simulink model "pwr_computeEnginePower"  (R2019b)
settings: Solver=FixedStepDiscrete  StartTime=0.0  StopTime=10.0  RelTol=1e-3
libraries: simulink x27
settings Model: Creator=vranken  LastModifiedBy=vranken
settings OptimizationCC: DefaultParameterBehavior=Inlined  EnhancedBackFolding=on  PassReuseOutputArgsAs=Individual arguments  ZeroExternalMemoryAtStartup=off  ZeroInternalMemoryAtStartup=off  OptimizeBlockOrder=speed  DifferentSizesBufferReuse=on  OptimizationCustomize=off  EfficientTunableParamExpr=on
settings DebuggingCC: ParameterTunabilityLossMsg=error
settings HardwareCC: ProdBitPerInt=16  ProdBitPerPointer=16  ProdBitPerSizeT=16  ProdBitPerPtrDiffT=16  ProdLargestAtomicFloat=None  ProdWordSize=8  ProdHWDeviceType=Atmel->AVR
settings SFSimCC: MATLABDynamicMemAlloc=off
settings RTWCC: SystemTargetFile=ert.tlc  GenCodeOnly=on  TemplateMakefile=ert_default_tmf  GenerateReport=on  IncludeHyperlinkInReport=on  LaunchReport=on  GenerateTraceInfo=on  GenerateTraceReport=on  GenerateTraceReportSl=on  GenerateTraceReportSf=on  GenerateTraceReportEml=on
settings CodeAppCC: ForceParamTrailComments=on  IgnoreCustomStorageClasses=off  OperatorAnnotations=on  SimulinkDataObjDesc=on  SFDataObjDesc=on  InsertBlockDesc=on
settings ERTTargetCC: TargetLangStandard=C99 (ISO)  SupportAbsoluteTime=off  PurelyIntegerCode=on  SupportNonFinite=off  SupportComplex=off  GenerateASAP2=on  InlinedParameterPlacement=NonHierarchical  ERTCustomFileTemplate=example_file_process.tlc  IndentStyle=Allman  IndentSize=4

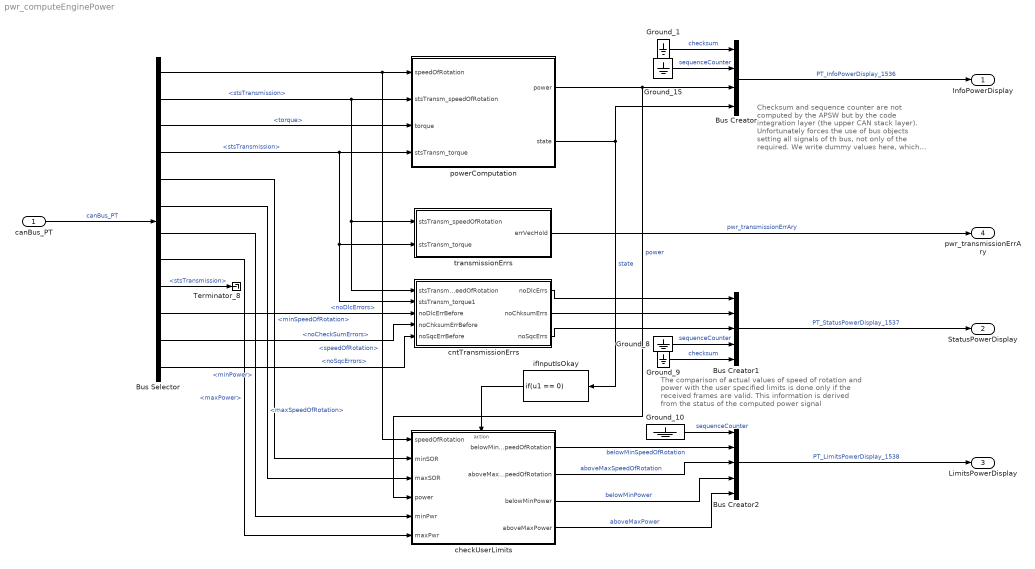
== system pwr_computeEnginePower ==
  note: The comparison of actual values of speed of rotation
      |  and power with the user specified limits is done only
      | if the received frames are valid. This information is
      | derived from the status of the computed power signal
  note: Checksum and sequence counter are not
      | computed by the APSW but by the code
      | integration layer (the upper CAN stack layer).
      | Unfortunately forces the use of bus objects
      | setting all signals of th bus, not only of
      | the required. We write dummy values here,
      | which will be overwritten by the CAN stack
  canBus_PT : Inport  OutDataTypeStr=Bus: cap_canBus_PT_t  BusOutputAsStruct=on
  Bus Creator : BusCreator  Inputs=4  OutDataTypeStr=Bus: cap_PT_InfoPowerDisplay_1536_t  NonVirtualBus=on
  Bus Creator1 : BusCreator  Inputs=5  OutDataTypeStr=Bus: cap_PT_StatusPowerDisplay_1537_t  NonVirtualBus=on
  Bus Creator2 : BusCreator  Inputs=5  OutDataTypeStr=Bus: cap_PT_LimitsPowerDisplay_1538_t  NonVirtualBus=on
  Bus Selector : BusSelector  OutputSignals=PT_StateEcu01_1024_sts.signals.speedOfRotation,PT_StateEcu01_1024_sts.stsTransmission,PT_StateEcu02_1040_sts.signals.torque,PT_StateEcu02_1040_sts.stsTransmission,PT_UserLimits_2032_sts.signals.minSpeedOfRotation,PT_UserLimits_2032_sts.signals.maxSpeedOfRotation,PT_UserLimits_2032_sts.signals.minPower,PT_UserLimits_2032_sts.signals.maxPower,PT_UserLimits_2032_sts.stsTransmission,PT_StatusPowerDisplay_1537_sts.signals.noDlcErrors,PT_StatusPowerDisplay_1537_sts.signals.noCheckSumErrors,PT_StatusPowerDisplay_1537_sts.signals.noSqcErrors
  Ground_{1,8..10,15} (5 alike) : Ground
  Terminator_8 : Terminator
  checkUserLimits : Subsystem  TreatAsAtomicUnit=on  RTWFcnName=pwr_detectAndCountError
      settings: RTWFcnNameOpts=User specified
  cntTransmissionErrs : Subsystem
  ifInputIsOkay : If  IfExpression=u1 == 0  ShowElse=off
  powerComputation : Subsystem
  transmissionErrs : Subsystem
  InfoPowerDisplay : Outport  OutDataTypeStr=Bus: cap_PT_InfoPowerDisplay_1536_t
  StatusPowerDisplay : Outport  Port=2  OutDataTypeStr=Bus: cap_PT_StatusPowerDisplay_1537_t
  LimitsPowerDisplay : Outport  Port=3  OutDataTypeStr=Bus: cap_PT_LimitsPowerDisplay_1538_t
  pwr_transmissionErrAry : Outport  Port=4
  wires:
  Bus Creator1/1 -> StatusPowerDisplay/1  "PT_StatusPowerDisplay_1537"
  Ground_15/1 -> Bus Creator/2  "sequenceCounter"
  Bus Selector/8 -> checkUserLimits/6(maxPwr)  "<maxPower>"
  Bus Selector/10 -> cntTransmissionErrs/3(noDlcErrBefore)  "<noDlcErrors>"
  Bus Selector/9 -> Terminator_8/1  "<stsTransmission>"
  Bus Selector/7 -> checkUserLimits/5(minPwr)  "<minPower>"
  powerComputation/1(power) -> Bus Creator/3, checkUserLimits/4(power)  "power"
  canBus_PT/1 -> Bus Selector/1  "canBus_PT"
  Bus Selector/6 -> checkUserLimits/3(maxSOR)  "<maxSpeedOfRotation>"
  powerComputation/2(state) -> Bus Creator/4, ifInputIsOkay/1  "state"
  cntTransmissionErrs/2(noChksumErrs) -> Bus Creator1/2
  ifInputIsOkay/1 -> checkUserLimits/Action
  Bus Selector/11 -> cntTransmissionErrs/4(noChksumErrBefore)  "<noCheckSumErrors>"
  Bus Selector/5 -> checkUserLimits/2(minSOR)  "<minSpeedOfRotation>"
  transmissionErrs/1(errVecHold) -> pwr_transmissionErrAry/1  "pwr_transmissionErrAry"
  Ground_1/1 -> Bus Creator/1  "checksum"
  checkUserLimits/4(aboveMaxPower) -> Bus Creator2/5  "aboveMaxPower"
  Bus Creator2/1 -> LimitsPowerDisplay/1  "PT_LimitsPowerDisplay_1538"
  cntTransmissionErrs/3(noSqcErrs) -> Bus Creator1/3
  Bus Selector/4 -> powerComputation/4(stsTransm_torque), cntTransmissionErrs/2(stsTransm_torque1), transmissionErrs/2(stsTransm_torque)  "<stsTransmission>"
  checkUserLimits/3(belowMinPower) -> Bus Creator2/4  "belowMinPower"
  Ground_9/1 -> Bus Creator1/5  "checksum"
  Bus Selector/1 -> powerComputation/1(speedOfRotation), checkUserLimits/1(speedOfRotation)  "<speedOfRotation>"
  checkUserLimits/2(aboveMaxSpeedOfRotation) -> Bus Creator2/3  "aboveMaxSpeedOfRotation"
  Bus Selector/3 -> powerComputation/3(torque)  "<torque>"
  cntTransmissionErrs/1(noDlcErrs) -> Bus Creator1/1
  Bus Selector/12 -> cntTransmissionErrs/5(noSqcErrBefore)  "<noSqcErrors>"
  Bus Selector/2 -> powerComputation/2(stsTransm_speedOfRotation), cntTransmissionErrs/1(stsTransm_speedOfRotation), transmissionErrs/1(stsTransm_speedOfRotation)  "<stsTransmission>"
  checkUserLimits/1(belowMinSpeedOfRotation) -> Bus Creator2/2  "belowMinSpeedOfRotation"
  Bus Creator/1 -> InfoPowerDisplay/1  "PT_InfoPowerDisplay_1536"
  Ground_8/1 -> Bus Creator1/4  "sequenceCounter"
  Ground_10/1 -> Bus Creator2/1  "sequenceCounter"

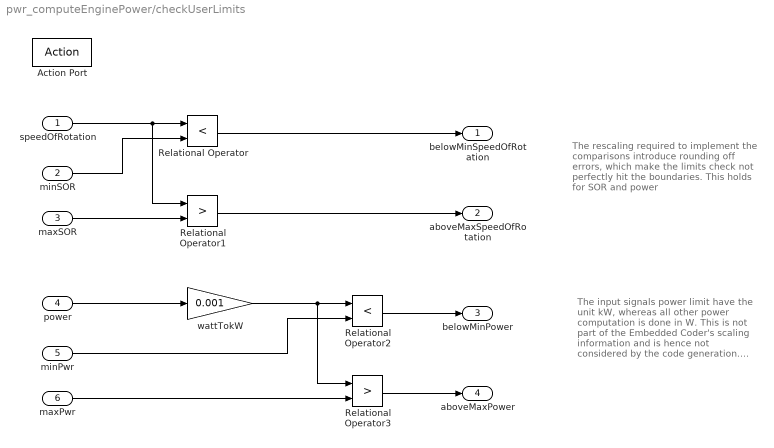
== system pwr_computeEnginePower/checkUserLimits ==
  note: The input signals power limit
      | have the unit kW, whereas all other
      | power computation is done in W.
      | This is not part of the Embedded
      | Coder's scaling information and is
      | hence not considered by the code
      | generation. We need to perform
      | this kind of rescaling by an explicit
      | multiplication operation
  note: The rescaling required to implement
      | the comparisons introduce rounding
      | off errors, which make the limits check
      | not perfectly hit the boundaries. This
      | holds for SOR and power
  speedOfRotation : Inport
  minSOR : Inport  Port=2
  maxSOR : Inport  Port=3
  power : Inport  Port=4
  minPwr : Inport  Port=5
  maxPwr : Inport  Port=6
  Action Port : ActionPort  PropagateVarSize=During execution  ActionPortLabel=if(u1 == 0)
  Relational Operator : RelationalOperator  Operator=<  OutDataTypeStr=boolean  RndMeth=Nearest
  Relational Operator1 : RelationalOperator  Operator=>  OutDataTypeStr=boolean  RndMeth=Nearest
  Relational Operator2 : RelationalOperator  Operator=<  OutDataTypeStr=boolean  RndMeth=Nearest
  Relational Operator3 : RelationalOperator  Operator=>  OutDataTypeStr=boolean  RndMeth=Nearest
  wattTokW : Gain  Gain=0.001  OutDataTypeStr=fixdt(0,16,2^-1,-10)
  belowMinSpeedOfRotation : Outport
  aboveMaxSpeedOfRotation : Outport  Port=2
  belowMinPower : Outport  Port=3
  aboveMaxPower : Outport  Port=4
  wires:
  speedOfRotation/1 -> Relational Operator/1, Relational Operator1/1
  minSOR/1 -> Relational Operator/2
  Relational Operator/1 -> belowMinSpeedOfRotation/1
  maxSOR/1 -> Relational Operator1/2
  Relational Operator1/1 -> aboveMaxSpeedOfRotation/1
  power/1 -> wattTokW/1
  minPwr/1 -> Relational Operator2/2
  Relational Operator2/1 -> belowMinPower/1
  maxPwr/1 -> Relational Operator3/2
  Relational Operator3/1 -> aboveMaxPower/1
  wattTokW/1 -> Relational Operator2/1, Relational Operator3/1

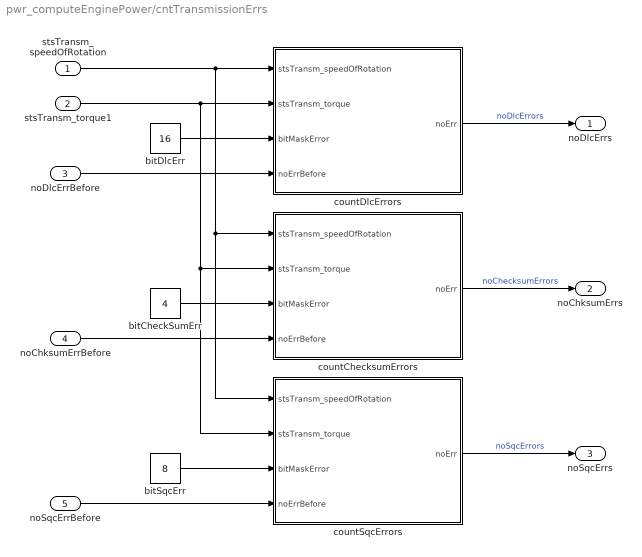
== system pwr_computeEnginePower/cntTransmissionErrs ==
  stsTransm_speedOfRotation : Inport
  stsTransm_torque1 : Inport  Port=2
  noDlcErrBefore : Inport  Port=3
  noChksumErrBefore : Inport  Port=4
  noSqcErrBefore : Inport  Port=5
  bitCheckSumErr : Constant  Value=4  OutDataTypeStr=uint8
  bitDlcErr : Constant  Value=16  OutDataTypeStr=uint8
  bitSqcErr : Constant  Value=8  OutDataTypeStr=uint8
  countChecksumErrors : Subsystem  TreatAsAtomicUnit=on  RTWFcnName=pwr_detectAndCountError
      settings: RTWFcnNameOpts=User specified
  countDlcErrors : Subsystem  TreatAsAtomicUnit=on  RTWFcnName=pwr_detectAndCountError
      settings: RTWFcnNameOpts=User specified
  countSqcErrors : Subsystem  TreatAsAtomicUnit=on  RTWFcnName=pwr_detectAndCountError
      settings: RTWFcnNameOpts=User specified
  noDlcErrs : Outport
  noChksumErrs : Outport  Port=2
  noSqcErrs : Outport  Port=3
  wires:
  bitDlcErr/1 -> countDlcErrors/3(bitMaskError)
  bitCheckSumErr/1 -> countChecksumErrors/3(bitMaskError)
  bitSqcErr/1 -> countSqcErrors/3(bitMaskError)
  stsTransm_speedOfRotation/1 -> countDlcErrors/1(stsTransm_speedOfRotation), countChecksumErrors/1(stsTransm_speedOfRotation), countSqcErrors/1(stsTransm_speedOfRotation)
  stsTransm_torque1/1 -> countDlcErrors/2(stsTransm_torque), countChecksumErrors/2(stsTransm_torque), countSqcErrors/2(stsTransm_torque)
  countDlcErrors/1(noErr) -> noDlcErrs/1  "noDlcErrors"
  noDlcErrBefore/1 -> countDlcErrors/4(noErrBefore)
  countChecksumErrors/1(noErr) -> noChksumErrs/1  "noChecksumErrors"
  noChksumErrBefore/1 -> countChecksumErrors/4(noErrBefore)
  countSqcErrors/1(noErr) -> noSqcErrs/1  "noSqcErrors"
  noSqcErrBefore/1 -> countSqcErrors/4(noErrBefore)

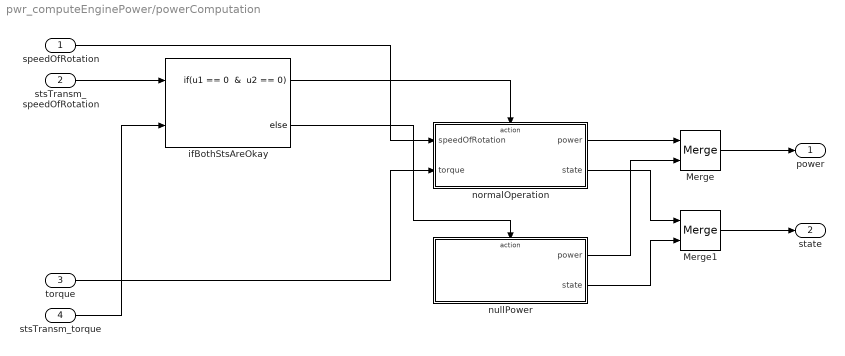
== system pwr_computeEnginePower/powerComputation ==
  speedOfRotation : Inport
  stsTransm_speedOfRotation : Inport  Port=2
  torque : Inport  Port=3
  stsTransm_torque : Inport  Port=4
  Merge : Merge
  Merge1 : Merge
  ifBothStsAreOkay : If  NumInputs=2  IfExpression="u1 == 0  &  u2 == 0"
  normalOperation : Subsystem  TreatAsAtomicUnit=on
  nullPower : Subsystem  TreatAsAtomicUnit=on
  power : Outport
  state : Outport  Port=2
  wires:
  speedOfRotation/1 -> normalOperation/1(speedOfRotation)
  stsTransm_speedOfRotation/1 -> ifBothStsAreOkay/1
  stsTransm_torque/1 -> ifBothStsAreOkay/2
  ifBothStsAreOkay/1 -> normalOperation/Action
  torque/1 -> normalOperation/2(torque)
  ifBothStsAreOkay/2 -> nullPower/Action
  normalOperation/1(power) -> Merge/1
  nullPower/1(power) -> Merge/2
  normalOperation/2(state) -> Merge1/1
  nullPower/2(state) -> Merge1/2
  Merge/1 -> power/1
  Merge1/1 -> state/1

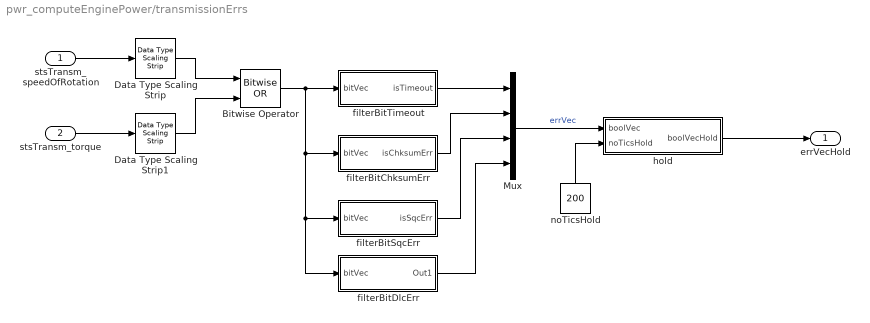
== system pwr_computeEnginePower/transmissionErrs ==
  stsTransm_speedOfRotation : Inport
  stsTransm_torque : Inport  Port=2
  Bitwise Operator : simulink/Logic and Bit Operations/Bitwise Operator  logicop=OR  UseBitMask=off  NumInputPorts=2  BitMask=bin2dec('11011001')  BitMaskRealWorld=Stored Integer
  Data Type Scaling Strip : simulink/Signal Attributes/Data Type Scaling Strip
      settings: SourceProductName=Simulink  SourceProductBaseCode=SL
  Data Type Scaling Strip1 : simulink/Signal Attributes/Data Type Scaling Strip
      settings: SourceProductName=Simulink  SourceProductBaseCode=SL
  Mux : Mux
  filterBitChksumErr : Subsystem
  filterBitDlcErr : Subsystem
  filterBitSqcErr : Subsystem
  filterBitTimeout : Subsystem
  hold : Subsystem
  noTicsHold : Constant  Value=200  OutDataTypeStr=uint8
  errVecHold : Outport
  wires:
  stsTransm_speedOfRotation/1 -> Data Type Scaling Strip/1
  stsTransm_torque/1 -> Data Type Scaling Strip1/1
  Data Type Scaling Strip/1 -> Bitwise Operator/1
  Mux/1 -> hold/1(boolVec)  "errVec"
  Data Type Scaling Strip1/1 -> Bitwise Operator/2
  Bitwise Operator/1 -> filterBitSqcErr/1(bitVec), filterBitDlcErr/1(bitVec), filterBitChksumErr/1(bitVec), filterBitTimeout/1(bitVec)
  filterBitChksumErr/1(isChksumErr) -> Mux/2
  filterBitSqcErr/1(isSqcErr) -> Mux/3
  filterBitDlcErr/1(Out1) -> Mux/4
  filterBitTimeout/1(isTimeout) -> Mux/1
  hold/1(boolVecHold) -> errVecHold/1
  noTicsHold/1 -> hold/2(noTicsHold)

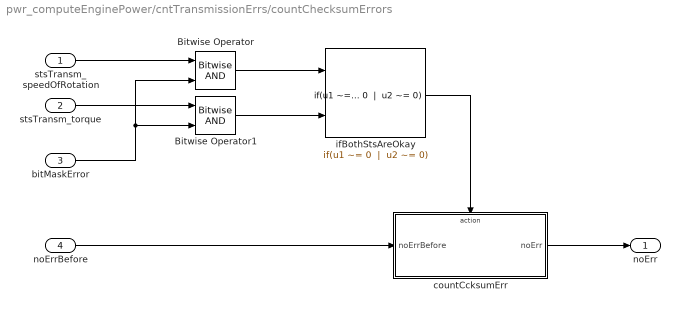
== system pwr_computeEnginePower/cntTransmissionErrs/countChecksumErrors ==
  stsTransm_speedOfRotation : Inport
  stsTransm_torque : Inport  Port=2
  bitMaskError : Inport  Port=3
  noErrBefore : Inport  Port=4
  Bitwise Operator : simulink/Logic and Bit Operations/Bitwise Operator  logicop=AND  UseBitMask=off  NumInputPorts=2  BitMask=bin2dec('11011001')  BitMaskRealWorld=Stored Integer
  Bitwise Operator1 : simulink/Logic and Bit Operations/Bitwise Operator  logicop=AND  UseBitMask=off  NumInputPorts=2  BitMask=bin2dec('11011001')  BitMaskRealWorld=Stored Integer
  countCcksumErr : Subsystem  TreatAsAtomicUnit=on
  ifBothStsAreOkay : If  NumInputs=2  IfExpression="u1 ~= 0  |  u2 ~= 0"  ShowElse=off
  noErr : Outport
  wires:
  ifBothStsAreOkay/1 -> countCcksumErr/Action
  stsTransm_torque/1 -> Bitwise Operator1/1
  stsTransm_speedOfRotation/1 -> Bitwise Operator/1
  noErrBefore/1 -> countCcksumErr/1(noErrBefore)
  countCcksumErr/1(noErr) -> noErr/1
  bitMaskError/1 -> Bitwise Operator/2, Bitwise Operator1/2
  Bitwise Operator/1 -> ifBothStsAreOkay/1
  Bitwise Operator1/1 -> ifBothStsAreOkay/2

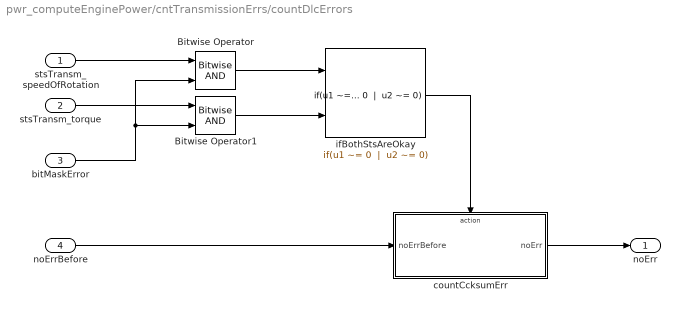
== system pwr_computeEnginePower/cntTransmissionErrs/countDlcErrors ==
  stsTransm_speedOfRotation : Inport
  stsTransm_torque : Inport  Port=2
  bitMaskError : Inport  Port=3
  noErrBefore : Inport  Port=4
  Bitwise Operator : simulink/Logic and Bit Operations/Bitwise Operator  logicop=AND  UseBitMask=off  NumInputPorts=2  BitMask=bin2dec('11011001')  BitMaskRealWorld=Stored Integer
  Bitwise Operator1 : simulink/Logic and Bit Operations/Bitwise Operator  logicop=AND  UseBitMask=off  NumInputPorts=2  BitMask=bin2dec('11011001')  BitMaskRealWorld=Stored Integer
  countCcksumErr : Subsystem  TreatAsAtomicUnit=on
  ifBothStsAreOkay : If  NumInputs=2  IfExpression="u1 ~= 0  |  u2 ~= 0"  ShowElse=off
  noErr : Outport
  wires:
  ifBothStsAreOkay/1 -> countCcksumErr/Action
  stsTransm_torque/1 -> Bitwise Operator1/1
  stsTransm_speedOfRotation/1 -> Bitwise Operator/1
  noErrBefore/1 -> countCcksumErr/1(noErrBefore)
  countCcksumErr/1(noErr) -> noErr/1
  bitMaskError/1 -> Bitwise Operator/2, Bitwise Operator1/2
  Bitwise Operator/1 -> ifBothStsAreOkay/1
  Bitwise Operator1/1 -> ifBothStsAreOkay/2

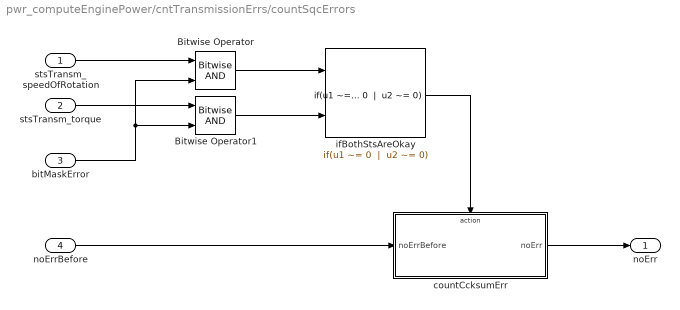
== system pwr_computeEnginePower/cntTransmissionErrs/countSqcErrors ==
  stsTransm_speedOfRotation : Inport
  stsTransm_torque : Inport  Port=2
  bitMaskError : Inport  Port=3
  noErrBefore : Inport  Port=4
  Bitwise Operator : simulink/Logic and Bit Operations/Bitwise Operator  logicop=AND  UseBitMask=off  NumInputPorts=2  BitMask=bin2dec('11011001')  BitMaskRealWorld=Stored Integer
  Bitwise Operator1 : simulink/Logic and Bit Operations/Bitwise Operator  logicop=AND  UseBitMask=off  NumInputPorts=2  BitMask=bin2dec('11011001')  BitMaskRealWorld=Stored Integer
  countCcksumErr : Subsystem  TreatAsAtomicUnit=on
  ifBothStsAreOkay : If  NumInputs=2  IfExpression="u1 ~= 0  |  u2 ~= 0"  ShowElse=off
  noErr : Outport
  wires:
  Bitwise Operator1/1 -> ifBothStsAreOkay/2
  Bitwise Operator/1 -> ifBothStsAreOkay/1
  bitMaskError/1 -> Bitwise Operator1/2, Bitwise Operator/2
  countCcksumErr/1(noErr) -> noErr/1
  noErrBefore/1 -> countCcksumErr/1(noErrBefore)
  stsTransm_speedOfRotation/1 -> Bitwise Operator/1
  stsTransm_torque/1 -> Bitwise Operator1/1
  ifBothStsAreOkay/1 -> countCcksumErr/Action

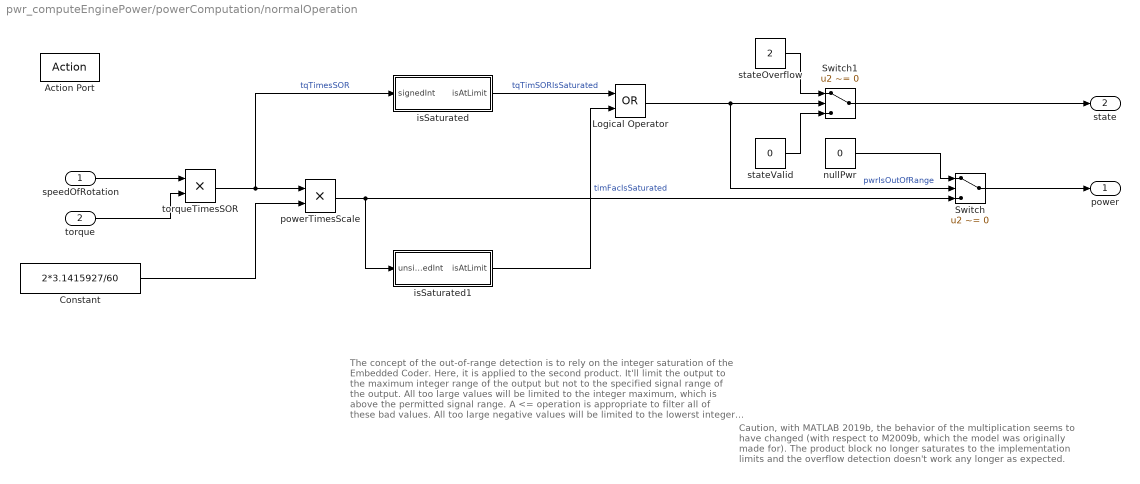
== system pwr_computeEnginePower/powerComputation/normalOperation ==
  note: Caution, with MATLAB 2019b, the behavior of the multiplication seems
      | to have changed (with respect to M2009b, which the model was
      | originally made for). The product block no longer saturates to the
      | implementation limits and the overflow detection doesn't work any
      | longer as expected.
  note: The concept of the out-of-range detection is to rely on the integer saturation
      | of the Embedded Coder. Here, it is applied to the second product. It'll limit
      | the output to the maximum integer range of the output but not to the specified
      | signal range of the output.
      |   All too large values will be limited to the integer maximum, which is above
      | the permitted signal range. A <= operation is appropriate to filter all of these
      | bad values.
      |   All too large negative values will be limited to the lowerst integer value, which
      | is the minimum permitted signal value at the same time. It's a binary zero. We
      | can't distinguish between a good but extreme value or a limited one if we see
      | the binary zero. This is ignored; binary zero is always considered a bad value.
      | Our logic effectively decreases the output signal range by one unit.
      |   A perfect out-of-range detection is nearly impossible in fixed point
      | computation since it requires some insight into the product operation. This
      | insight does the EC have during code generation but we don't have it on the
      | Simulink level.
      |  The best compromise would be the rule to never include the largest and
      | lowest integer values in the permitted signal range - then a safe detection
      | becomes possible in the way we present it here
  speedOfRotation : Inport
  torque : Inport  Port=2
  Action Port : ActionPort  PropagateVarSize=During execution  ActionPortLabel="if(u1 == 0  &  u2 == 0)"
  Constant : Constant  Value=2*3.1415927/60  OutDataTypeStr=fixdt(0,16,19)
  Logical Operator : Logic  Operator=OR  AllPortsSameDT=off  OutDataTypeStr=boolean
  Switch : Switch  Criteria=u2 ~= 0  OutDataTypeStr=Inherit: Inherit via back propagation
  Switch1 : Switch  Criteria=u2 ~= 0  OutDataTypeStr=Inherit: Inherit via back propagation
  isSaturated : Subsystem
  isSaturated1 : Subsystem
  nullPwr : Constant  Value=0  OutDataTypeStr=Inherit: Inherit via back propagation
  powerTimesScale : Product  OutDataTypeStr=fixdt(0,16,2^5,-500000)  RndMeth=Simplest  SaturateOnIntegerOverflow=on
  stateOverflow : Constant  Value=2  OutDataTypeStr=uint8
  stateValid : Constant  Value=0  OutDataTypeStr=uint8
  torqueTimesSOR : Product  OutMin=6553.5*(-500)  OutMax=6553.5*500  OutDataTypeStr=fixdt(1,32,9)  RndMeth=Simplest  SaturateOnIntegerOverflow=on
  power : Outport  InitialOutput=0
  state : Outport  Port=2  InitialOutput=1
  wires:
  speedOfRotation/1 -> torqueTimesSOR/1
  torque/1 -> torqueTimesSOR/2
  Constant/1 -> powerTimesScale/2
  powerTimesScale/1 -> isSaturated1/1(unsignedInt), Switch/3
  Switch/1 -> power/1
  Logical Operator/1 -> Switch1/2, Switch/2  "pwrIsOutOfRange"
  stateOverflow/1 -> Switch1/1
  stateValid/1 -> Switch1/3
  Switch1/1 -> state/1
  torqueTimesSOR/1 -> powerTimesScale/1, isSaturated/1(signedInt)  "tqTimesSOR"
  isSaturated/1(isAtLimit) -> Logical Operator/1  "tqTimSORIsSaturated"
  isSaturated1/1(isAtLimit) -> Logical Operator/2  "timFacIsSaturated"
  nullPwr/1 -> Switch/1

== system pwr_computeEnginePower/powerComputation/nullPower ==
  Action Port : ActionPort  PropagateVarSize=During execution  ActionPortLabel=else
  Constant : Constant  Value=0  OutDataTypeStr=Inherit: Inherit via back propagation
  stateInvalidInput : Constant  OutDataTypeStr=uint8
  power : Outport  InitialOutput=0
  state : Outport  Port=2  InitialOutput=1
  wires:
  Constant/1 -> power/1
  stateInvalidInput/1 -> state/1

== system pwr_computeEnginePower/transmissionErrs/filterBitChksumErr ==
  bitVec : Inport
  Compare To Zero : simulink/Logic and Bit Operations/Compare To Zero  relop=~=  OutDataTypeStr=boolean  ZeroCross=off
  andBitChksumErr : simulink/Logic and Bit Operations/Bitwise Operator  logicop=AND  UseBitMask=on  BitMask=4  BitMaskRealWorld=Stored Integer
  isChksumErr : Outport
  wires:
  bitVec/1 -> andBitChksumErr/1
  andBitChksumErr/1 -> Compare To Zero/1
  Compare To Zero/1 -> isChksumErr/1  "isChksumErr"

== system pwr_computeEnginePower/transmissionErrs/filterBitDlcErr ==
  bitVec : Inport
  Compare To Zero : simulink/Logic and Bit Operations/Compare To Zero  relop=~=  OutDataTypeStr=boolean  ZeroCross=off
  andBitDlcErr : simulink/Logic and Bit Operations/Bitwise Operator  logicop=AND  UseBitMask=on  BitMask=16  BitMaskRealWorld=Stored Integer
  Out1 : Outport
  wires:
  bitVec/1 -> andBitDlcErr/1
  andBitDlcErr/1 -> Compare To Zero/1
  Compare To Zero/1 -> Out1/1  "isDlcErr"

== system pwr_computeEnginePower/transmissionErrs/filterBitSqcErr ==
  note: isSqcErr
  bitVec : Inport
  Compare To Zero : simulink/Logic and Bit Operations/Compare To Zero  relop=~=  OutDataTypeStr=boolean  ZeroCross=off
  andBitSqcErr : simulink/Logic and Bit Operations/Bitwise Operator  logicop=AND  UseBitMask=on  BitMask=8  BitMaskRealWorld=Stored Integer
  isSqcErr : Outport
  wires:
  bitVec/1 -> andBitSqcErr/1
  andBitSqcErr/1 -> Compare To Zero/1
  Compare To Zero/1 -> isSqcErr/1

== system pwr_computeEnginePower/transmissionErrs/filterBitTimeout ==
  bitVec : Inport
  Compare To Zero : simulink/Logic and Bit Operations/Compare To Zero  relop=~=  OutDataTypeStr=boolean  ZeroCross=off
  andBitTimeout : simulink/Logic and Bit Operations/Bitwise Operator  logicop=AND  UseBitMask=on  BitMask=2  BitMaskRealWorld=Stored Integer
  isTimeout : Outport
  wires:
  andBitTimeout/1 -> Compare To Zero/1  "errTimeout"
  bitVec/1 -> andBitTimeout/1
  Compare To Zero/1 -> isTimeout/1  "isTimeout"

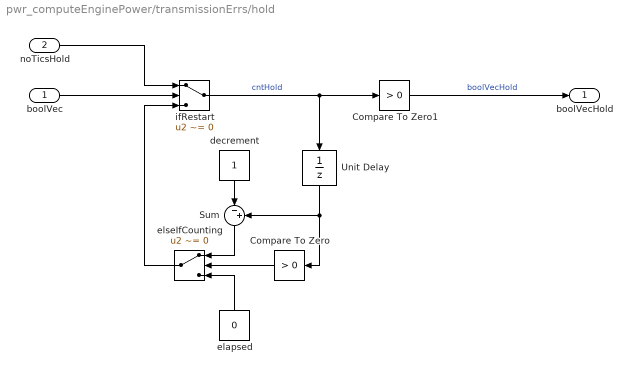
== system pwr_computeEnginePower/transmissionErrs/hold ==
  boolVec : Inport
  noTicsHold : Inport  Port=2
  Compare To Zero : simulink/Logic and Bit Operations/Compare To Zero  relop=>  OutDataTypeStr=boolean  ZeroCross=off
  Compare To Zero1 : simulink/Logic and Bit Operations/Compare To Zero  relop=>  OutDataTypeStr=boolean  ZeroCross=off
  Sum : Sum  Inputs=|-+
  Unit Delay : UnitDelay  SampleTime=-1
  decrement : Constant  OutDataTypeStr=uint8
  elapsed : Constant  Value=0  OutDataTypeStr=uint8
  elseIfCounting : Switch  Criteria=u2 ~= 0
  ifRestart : Switch  Criteria=u2 ~= 0
  boolVecHold : Outport
  wires:
  noTicsHold/1 -> ifRestart/1
  Unit Delay/1 -> Sum/2, Compare To Zero/1
  Sum/1 -> elseIfCounting/1
  decrement/1 -> Sum/1
  elapsed/1 -> elseIfCounting/3
  ifRestart/1 -> Unit Delay/1, Compare To Zero1/1  "cntHold"
  elseIfCounting/1 -> ifRestart/3
  Compare To Zero/1 -> elseIfCounting/2
  Compare To Zero1/1 -> boolVecHold/1  "boolVecHold"
  boolVec/1 -> ifRestart/2

== system pwr_computeEnginePower/cntTransmissionErrs/countChecksumErrors/countCcksumErr ==
  noErrBefore : Inport
  Action Port : ActionPort  PropagateVarSize=During execution  ActionPortLabel="if(u1 ~= 0  |  u2 ~= 0)"
  Sum : Sum  Inputs=|++
  increment : Constant  OutDataTypeStr=uint8
  noErr : Outport
  wires:
  noErrBefore/1 -> Sum/1
  Sum/1 -> noErr/1  "noChecksumErrors"
  increment/1 -> Sum/2

== system pwr_computeEnginePower/cntTransmissionErrs/countDlcErrors/countCcksumErr ==
  noErrBefore : Inport
  Action Port : ActionPort  PropagateVarSize=During execution  ActionPortLabel="if(u1 ~= 0  |  u2 ~= 0)"
  Sum : Sum  Inputs=|++
  increment : Constant  OutDataTypeStr=uint8
  noErr : Outport
  wires:
  noErrBefore/1 -> Sum/1
  Sum/1 -> noErr/1  "noDlcErrors"
  increment/1 -> Sum/2

== system pwr_computeEnginePower/cntTransmissionErrs/countSqcErrors/countCcksumErr ==
  noErrBefore : Inport
  Action Port : ActionPort  PropagateVarSize=During execution  ActionPortLabel="if(u1 ~= 0  |  u2 ~= 0)"
  Sum : Sum  Inputs=|++
  increment : Constant  OutDataTypeStr=uint8
  noErr : Outport
  wires:
  increment/1 -> Sum/2
  Sum/1 -> noErr/1  "noSqcErrors"
  noErrBefore/1 -> Sum/1

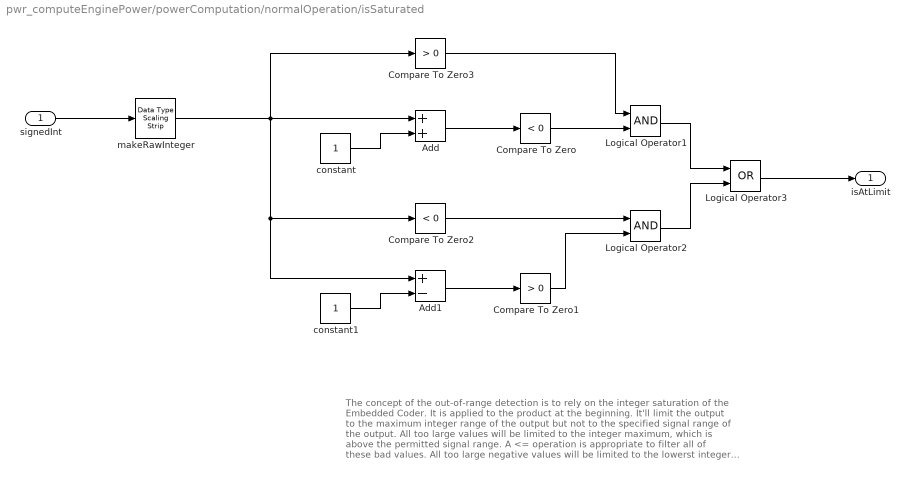
== system pwr_computeEnginePower/powerComputation/normalOperation/isSaturated ==
  note: The concept of the out-of-range detection is to rely on the integer saturation
      | of the Embedded Coder. It is applied to the product at the beginning. It'll limit
      | the output to the maximum integer range of the output but not to the specified
      | signal range of the output.
      |   All too large values will be limited to the integer maximum, which is above
      | the permitted signal range. A <= operation is appropriate to filter all of these
      | bad values.
      |   All too large negative values will be limited to the lowerst integer value, which
      | is the minimum permitted signal value at the same time. It's a binary zero. We
      | can't distinguish between a good but extreme value or a limited one if we see
      | the binary zero. This is ignored; binary zero is always considered a bad value.
      | Our logic effectively decreases the output signal range by one unit.
      |   A perfect out-of-range detection is nearly impossible in fixed point
      | computation since it requires some insight into the product operation. This
      | insight does the EC have during code generation but we don't have it on the
      | Simulink level.
      |  The best compromise would be the rule to never include the largest and
      | lowest integer values in the permitted signal range - then a safe detection
      | becomes possible in the way we present it here
  signedInt : Inport
  Add : Sum  OutDataTypeStr=Inherit: Same as accumulator  RndMeth=Simplest
  Add1 : Sum  Inputs=+-  OutDataTypeStr=Inherit: Same as accumulator  RndMeth=Simplest
  Compare To Zero : simulink/Logic and Bit Operations/Compare To Zero  relop=<  OutDataTypeStr=boolean  ZeroCross=off
  Compare To Zero1 : simulink/Logic and Bit Operations/Compare To Zero  relop=>  OutDataTypeStr=boolean  ZeroCross=off
  Compare To Zero2 : simulink/Logic and Bit Operations/Compare To Zero  relop=<  OutDataTypeStr=boolean  ZeroCross=off
  Compare To Zero3 : simulink/Logic and Bit Operations/Compare To Zero  relop=>  OutDataTypeStr=boolean  ZeroCross=off
  Logical Operator1 : Logic  AllPortsSameDT=off  OutDataTypeStr=boolean
  Logical Operator2 : Logic  AllPortsSameDT=off  OutDataTypeStr=boolean
  Logical Operator3 : Logic  Operator=OR  AllPortsSameDT=off  OutDataTypeStr=boolean
  constant : Constant  OutDataTypeStr=Inherit: Inherit via back propagation
  constant1 : Constant  OutDataTypeStr=Inherit: Inherit via back propagation
  makeRawInteger : simulink/Signal Attributes/Data Type Scaling Strip
      settings: SourceProductName=Simulink  SourceProductBaseCode=SL
  isAtLimit : Outport
  wires:
  constant/1 -> Add/2
  signedInt/1 -> makeRawInteger/1
  Add/1 -> Compare To Zero/1
  constant1/1 -> Add1/2
  Add1/1 -> Compare To Zero1/1
  Compare To Zero2/1 -> Logical Operator2/1
  Compare To Zero1/1 -> Logical Operator2/2
  Compare To Zero3/1 -> Logical Operator1/1
  Compare To Zero/1 -> Logical Operator1/2
  Logical Operator1/1 -> Logical Operator3/1
  Logical Operator2/1 -> Logical Operator3/2
  Logical Operator3/1 -> isAtLimit/1
  makeRawInteger/1 -> Add/1, Add1/1, Compare To Zero2/1, Compare To Zero3/1

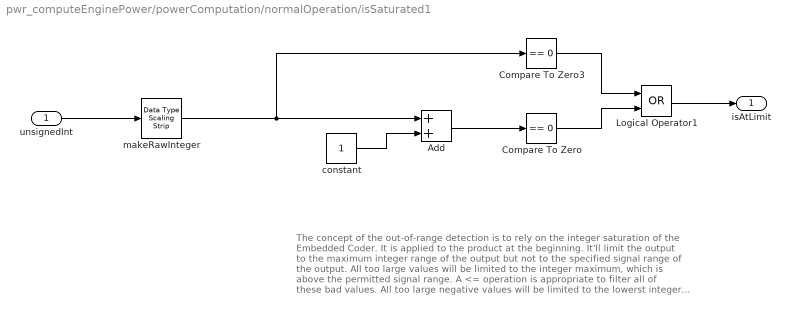
== system pwr_computeEnginePower/powerComputation/normalOperation/isSaturated1 ==
  note: The concept of the out-of-range detection is to rely on the integer saturation
      | of the Embedded Coder. It is applied to the product at the beginning. It'll limit
      | the output to the maximum integer range of the output but not to the specified
      | signal range of the output.
      |   All too large values will be limited to the integer maximum, which is above
      | the permitted signal range. A <= operation is appropriate to filter all of these
      | bad values.
      |   All too large negative values will be limited to the lowerst integer value, which
      | is the minimum permitted signal value at the same time. It's a binary zero. We
      | can't distinguish between a good but extreme value or a limited one if we see
      | the binary zero. This is ignored; binary zero is always considered a bad value.
      | Our logic effectively decreases the output signal range by one unit.
      |   A perfect out-of-range detection is nearly impossible in fixed point
      | computation since it requires some insight into the product operation. This
      | insight does the EC have during code generation but we don't have it on the
      | Simulink level.
      |  The best compromise would be the rule to never include the largest and
      | lowest integer values in the permitted signal range - then a safe detection
      | becomes possible in the way we present it here
  unsignedInt : Inport
  Add : Sum  OutDataTypeStr=Inherit: Same as accumulator  RndMeth=Simplest
  Compare To Zero : simulink/Logic and Bit Operations/Compare To Zero  relop===  OutDataTypeStr=boolean  ZeroCross=off
  Compare To Zero3 : simulink/Logic and Bit Operations/Compare To Zero  relop===  OutDataTypeStr=boolean  ZeroCross=off
  Logical Operator1 : Logic  Operator=OR  AllPortsSameDT=off  OutDataTypeStr=boolean
  constant : Constant  OutDataTypeStr=Inherit: Inherit via back propagation
  makeRawInteger : simulink/Signal Attributes/Data Type Scaling Strip
      settings: SourceProductName=Simulink  SourceProductBaseCode=SL
  isAtLimit : Outport
  wires:
  makeRawInteger/1 -> Compare To Zero3/1, Add/1
  Logical Operator1/1 -> isAtLimit/1
  Compare To Zero/1 -> Logical Operator1/2
  Compare To Zero3/1 -> Logical Operator1/1
  Add/1 -> Compare To Zero/1
  unsignedInt/1 -> makeRawInteger/1
  constant/1 -> Add/2
